simulink model "No_Kalman_FullSystem"  (R2024a)
settings: Solver=FixedStepAuto  StartTime=0.0  StopTime=0.05  FixedStep=0.05  RelTol=1e-3
model workspace (MAT data in the model file):
  Delta_t = 0.1
  J1 = 0.833333333333
  J2 = 1.08333333333
  J3 = 0.416666666667
  NoiseCov = [0.5  0  0  0  0  0  0; 0  0.5  0  0  0  0  0; 0  0  0.5  0  0  0  0; 0  0  0  0.5  0  0  0; 0  0  0  0  0.5  0  0; 0  0  0  0  0  0.5  0; 0  0  0  0  0  0  0.5]
  Orbit_Incl = 51.6
  Q_identity = [0.05  0  0  0  0  0  0; 0  0.05  0  0  0  0  0; 0  0  0.05  0  0  0  0; 0  0  0  0.05  0  0  0; 0  0  0  0  0.05  0  0; 0  0  0  0  0  0.05  0; 0  0  0  0  0  0  0.05]
  Sig = Simulink.Signal
  Sig.DataType = 'auto'
  Sig.Dimensions = -1
  Sig.DimensionsMode = 'auto'
  Sig.Complexity = 'auto'
  Sig.SampleTime = -1
  Sig.SamplingMode = 'auto'
  controlRun = 1
  jd_input = 2458850.00006
  m = 100
  n = 7
  prev_torque_input = [-0.00050779436613; -0.000537657150204; 0.000673104501962]
  q_ff_in = [0.768162333731 -0.000607721012165 0.00073835510125 -0.64025441392]
  s_input = [0.126195549094  -0.0456814887308  -0.161020672839  -0.0555064713506  -0.000532606081941  0.000213749478451  -0.00066383496662; -0.0456814887308  0.0300852731757  0.0643242310821  0.0221411903621  0.000189759589489  -0.00017191746789  0.000231570257692; -0.161020672839  0.0643242310821  0.23849220968  0.0781228177648  0.000857803282785  -0.000316346290687  0.000810872548691; -0.0555064713506  0.0221411903621  0.0781228177648  0.0387660028181  0.000267247923751  -0.000128314700029  0.000266373914183; -0.000532606081941  0.000189759589489  0.000857803282785  0.000267247923751  0.0414168924362  -1.57036491515e-05  2.42567511858e-05; 0.000213749478451  -0.00017191746789  -0.000316346290687  -0.000128314700029  -1.57036491515e-05  0.0414098493382  -0.000222921548759; -0.00066383496662  0.000231570257692  0.000810872548691  0.000266373914183  2.42567511858e-05  -0.000222921548759  0.0414237557466]
  s_input_cons = [1.94870414  1.25588909  1.4416761  1.0780205  1.49168854  1.53894753  1.37981514; 1.25588909  2.30599344  1.57766712  1.62980068  1.46050557  1.31460547  1.13813509; 1.4416761  1.57766712  1.70958392  1.12140846  1.38322267  1.58836736  1.34392315; 1.0780205  1.62980068  1.12140846  1.77837393  1.21690337  0.94427956  1.46043147; 1.49168854  1.46050557  1.38322267  1.21690337  2.06327445  1.39185931  1.33424815; 1.53894753  1.31460547  1.58836736  0.94427956  1.39185931  2.02772691  1.7277207; 1.37981514  1.13813509  1.34392315  1.46043147  1.33424815  1.7277207  2.16380015]
  savedTorque = [-0.000405741986708; 0.000253632743324; 0.00087809103841]
  t_step = 0.05
  v_icrf_input = [-2750.79951667 6666.40019935 2573.40073342]
  x_icrf_input = [3649696.21765 3308209.1663 -4676596.46157]
  x_icrf_input_cons = [3649700 3308200 -4676600]
  x_input = [-0.400194557056; -0.190242708716; -0.896104173464; -0.0254821228337; 0.443902714712; -0.277487336755; -0.960677002834]
  x_input_cons = [0.2; 0.6; 0.5; 0.59160797831; 0.1; 0.4; 0.9]
libraries: aerolibsatdyn x1, aerolibtransform2 x1, aerolibutil x1
settings Model: Creator=alenachan  LastModifiedBy=ruimi

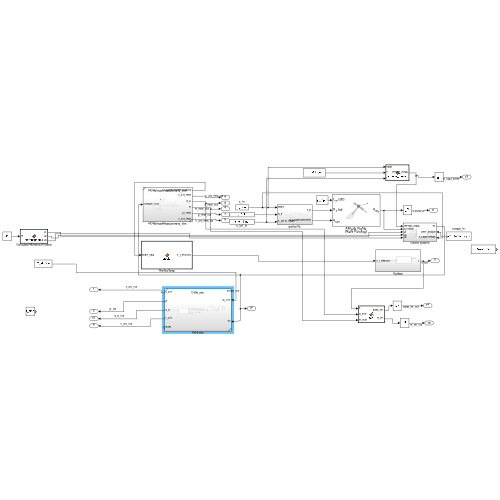
[thumbnail: Simulink's stored preview of the top-level diagram]
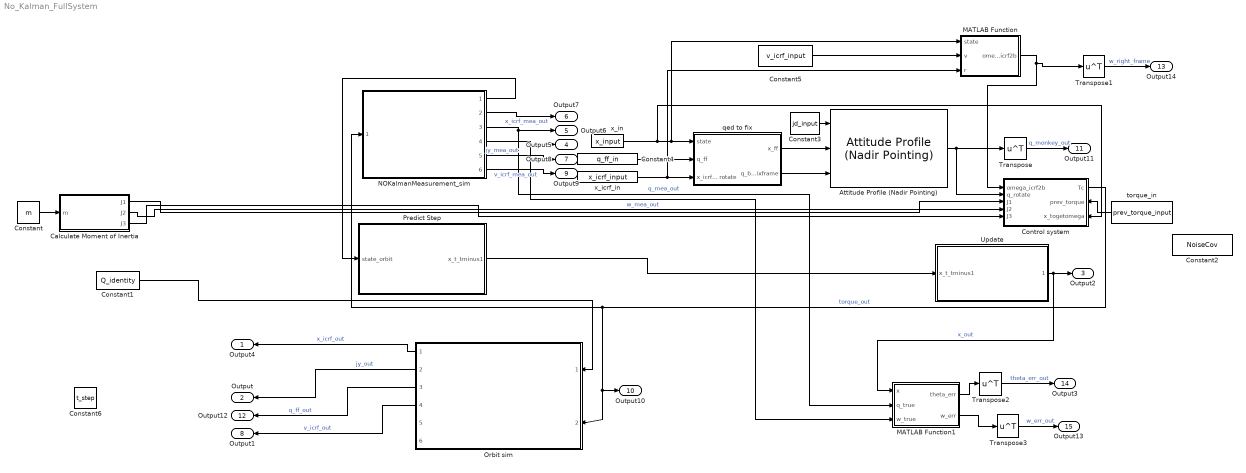
== system No_Kalman_FullSystem ==
  " Calculate Moment of Inertia" : MATLAB Function  Priority=10  TreatAsAtomicUnit=on
  Attitude Profile (Nadir Pointing) : aerolibsatdyn/Attitude Profile (Nadir Pointing)  Priority=3  outputError=on  outputFinalAttitude=off  portFrame=Fixed-frame  pointingMode=Point at nadir  celestialTarget=Sun  tunablePointing=off  primaryAlignmentSrc=Dialog  primaryAlignment=[0 0 1]  secondaryAlignmentSrc=Dialog  secondaryAlignment=[1 0 0]  constraintFrame=ICRF  primaryConstraintSrc=Dialog  primaryConstraint=[1 0 0]  secondaryConstraintSrc=Dialog  secondaryConstraint=[0 1 0]
  Constant : Constant  Value=m
  Constant1 : Constant  Value=Q_identity
  Constant2 : Constant  Value=NoiseCov
  Constant3 : Constant  Value=jd_input
  Constant4 : Constant  Value=q_ff_in
  Constant5 : Constant  Value=v_icrf_input
  Constant6 : Constant  Value=t_step
  Control system : Subsystem  Priority=4
      settings: PortSchema="{\"entries\":[{\"content\":{\"sides\":[{\"content\":{\"connectorIds\":[\"In1\",\"In2\",\"In3\",\"In4\",\"In5\"]},\"type\":\"ConnectorPlacement.EquallySpacedRectSide\",\"uuid\":\"8eb5f269-cc65-4267-936a-9f0f4ccd4d18\"},{\"content\":{\"connectorIds\":[\"Out1\",\"In6\",\"In7\"],\"side\":\"RIGHT\"},\"type\":\"ConnectorPlacement.EquallySpacedRectSide\",\"uuid\":\"3df96c14-e4ae-45ba-8fc0-de3a9fdcf55a\"},{\"content\":{\"side\":\"TOP\"},\"type\":\"ConnectorPlacement.EquallySpacedRectSide\",\"uuid\":\"e3effbcc-2fcc-4dea-811c-5aa639521533\"}]},\"type\":\"ConnectorPlacement.EquallySpacedConnector\",\"uuid\":\"93bbc224-b85a-4291-8bf8-2645c40efc9b\"}],\"packageUris\":[\"http://schema.mathworks.com/mf0/Connector/R2020b\"],\"version\":\"1.0\"}"
  MATLAB Function : MATLAB Function  TreatAsAtomicUnit=on
  MATLAB Function1 : MATLAB Function  TreatAsAtomicUnit=on
  NOKalmanMeasurement_sim : Subsystem  ReferencedSubsystem=NOKalmanMeasurement_sim
  Orbit sim : Subsystem  Priority=7  ReferencedSubsystem=Orbit_sim
  Predict Step : MATLAB Function  Priority=11  TreatAsAtomicUnit=on
  Transpose{,1..3} (4 alike) : Math  Operator=transpose
  Update : Subsystem  Priority=12
  qed to fix : Subsystem  Priority=2
  torque_in : Constant  Value=prev_torque_input
  x_icrf_in : Constant  Value=x_icrf_input
  x_in : Constant  Value=x_input
  Output4 : Outport
  Output : Outport  Port=2
  Output2 : Outport  Port=3
  Output5 : Outport  Port=4
  Output6 : Outport  Port=5
  Output7 : Outport  Port=6
  Output8 : Outport  Port=7
  Output1 : Outport  Port=8
  Output9 : Outport  Port=9
  Output10 : Outport  Port=10
  Output11 : Outport  Port=11
  Output12 : Outport  Port=12
  Output14 : Outport  Port=13
  Output3 : Outport  Port=14
  Output13 : Outport  Port=15
  wires:
  Control system/1(Tc) -> NOKalmanMeasurement_sim/1, Output10/1, Orbit sim/2  "torque_out"
  Orbit sim/2 -> Output/1  "jy_out"
  Orbit sim/1 -> Output4/1  "x_icrf_out"
  Constant/1 -> " Calculate Moment of Inertia"/1(m)
  " Calculate Moment of Inertia"/1(J1) -> Control system/3(J1)
  " Calculate Moment of Inertia"/2(J2) -> Control system/4(J2)
  " Calculate Moment of Inertia"/3(J3) -> Control system/5(J3)
  Constant1/1 -> Orbit sim/1
  x_in/1 -> Control system/7(x_togetomega), MATLAB Function/1(state), qed to fix/1(state)
  x_icrf_in/1 -> MATLAB Function/3(r), qed to fix/3(x_icrf to rotate)
  Predict Step/1(x_t_tminus1) -> Update/1(x_t_tminus1)
  Update/1(1) -> MATLAB Function1/1(x), Output2/1  "x_out"
  Orbit sim/3 -> Output12/1  "q_ff_out"
  NOKalmanMeasurement_sim/4 -> MATLAB Function1/3(w_true), Output5/1  "w_mea_out"
  NOKalmanMeasurement_sim/3 -> MATLAB Function1/2(q_true), Output6/1  "q_mea_out"
  NOKalmanMeasurement_sim/2 -> Output7/1  "x_icrf_mea_out"
  NOKalmanMeasurement_sim/5 -> Output8/1  "jy_mea_out"
  Orbit sim/4 -> Output1/1  "v_icrf_out"
  NOKalmanMeasurement_sim/6 -> Output9/1  "v_icrf_mea_out"
  torque_in/1 -> Control system/6(prev_torque)
  Transpose/1 -> Output11/1  "q_monkey_out"
  Constant3/1 -> Attitude Profile (Nadir Pointing)/1
  qed to fix/2(q_bodyToFixframe) -> Attitude Profile (Nadir Pointing)/3
  Constant4/1 -> qed to fix/2(q_ff)
  qed to fix/1(x_ff) -> Attitude Profile (Nadir Pointing)/2
  Attitude Profile (Nadir Pointing)/1 -> Transpose/1, Control system/2(q_rotate)
  Constant5/1 -> MATLAB Function/2(v)
  MATLAB Function/1(omega_icrf2b) -> Transpose1/1, Control system/1(omega_icrf2b)
  Transpose1/1 -> Output14/1  "w_right_frame"
  NOKalmanMeasurement_sim/1 -> Predict Step/1(state_orbit)
  MATLAB Function1/1(theta_err) -> Transpose2/1
  Transpose2/1 -> Output3/1  "theta_err_out"
  MATLAB Function1/2(w_err) -> Transpose3/1
  Transpose3/1 -> Output13/1  "w_err_out"

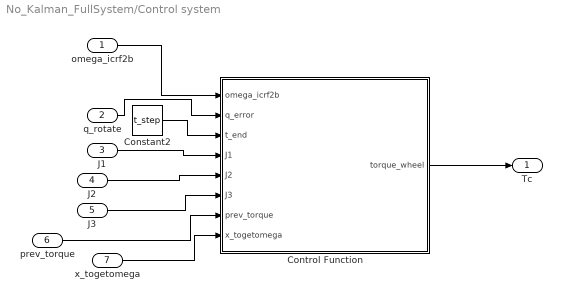
== system No_Kalman_FullSystem/Control system ==
  omega_icrf2b : Inport
  q_rotate : Inport  Port=2
  J1 : Inport  Port=3
  J2 : Inport  Port=4
  J3 : Inport  Port=5
  prev_torque : Inport  Port=6
  x_togetomega : Inport  Port=7
  Constant2 : Constant  Value=t_step
  Control Function : MATLAB Function  TreatAsAtomicUnit=on
  Tc : Outport
  wires:
  Constant2/1 -> Control Function/3(t_end)
  Control Function/1(torque_wheel) -> Tc/1
  q_rotate/1 -> Control Function/2(q_error)
  J1/1 -> Control Function/4(J1)
  J2/1 -> Control Function/5(J2)
  J3/1 -> Control Function/6(J3)
  prev_torque/1 -> Control Function/7(prev_torque)
  x_togetomega/1 -> Control Function/8(x_togetomega)
  omega_icrf2b/1 -> Control Function/1(omega_icrf2b)

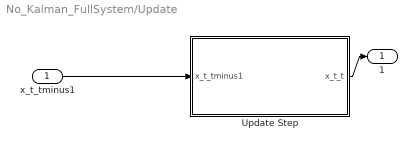
== system No_Kalman_FullSystem/Update ==
  x_t_tminus1 : Inport
  Update Step : MATLAB Function  TreatAsAtomicUnit=on
  1 : Outport
  wires:
  x_t_tminus1/1 -> Update Step/1(x_t_tminus1)
  Update Step/1(x_t_t) -> 1/1

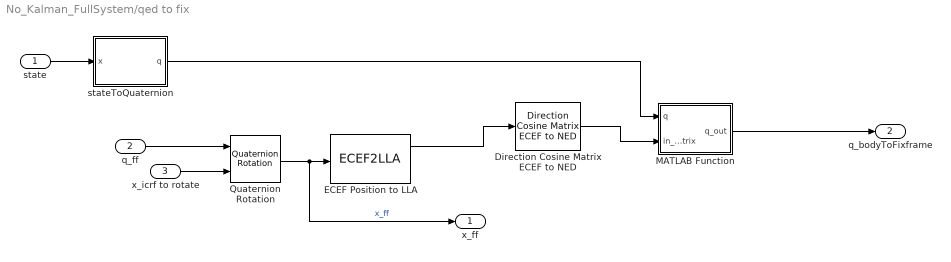
== system No_Kalman_FullSystem/qed to fix ==
  state : Inport
  q_ff : Inport  Port=2
  x_icrf to rotate : Inport  Port=3
  Direction Cosine Matrix ECEF to NED : aerolibtransform2/Direction Cosine Matrix ECEF to NED
  ECEF Position to LLA : ECEF2LLA
  MATLAB Function : MATLAB Function  TreatAsAtomicUnit=on
  Quaternion Rotation : aerolibutil/Quaternion Rotation
  stateToQuaternion : MATLAB Function  TreatAsAtomicUnit=on
  x_ff : Outport
  q_bodyToFixframe : Outport  Port=2
  wires:
  state/1 -> stateToQuaternion/1(x)
  Quaternion Rotation/1 -> x_ff/1, ECEF Position to LLA/1  "x_ff"
  x_icrf to rotate/1 -> Quaternion Rotation/2
  ECEF Position to LLA/1 -> Direction Cosine Matrix ECEF to NED/1
  Direction Cosine Matrix ECEF to NED/1 -> MATLAB Function/2(in_matrix)
  stateToQuaternion/1(q) -> MATLAB Function/1(q)
  MATLAB Function/1(q_out) -> q_bodyToFixframe/1
  q_ff/1 -> Quaternion Rotation/1

== matlab function No_Kalman_FullSystem/Update/Update Step ==
  data: x_t_tminus1 input; x_t_t output
function x_t_t  = update(x_t_tminus1)

%Update
x_t_t = x_t_tminus1;
x_t_t(1:4)=x_t_t(1:4)/norm(x_t_t(1:4));

end

== matlab function No_Kalman_FullSystem/Predict Step ==
  data: state_orbit input; x_t_tminus1 output
function x_t_tminus1 = predict(state_orbit)


x_t_tminus1 = state_orbit; %use state from orbit with noise
% x_t_tminus1 = feval(f_t,x_tminus1_tminus1);

== matlab function No_Kalman_FullSystem/qed to fix/MATLAB Function ==
  data: q input; in_matrix input; q_out output
function q_out= fcn(q, in_matrix)
inv_m = inv(in_matrix);
q_second = rotm2quat(inv_m);
q_first = quatconj(q);
q_out = transpose(quatmultiply(q_second,q_first));

== matlab function No_Kalman_FullSystem/qed to fix/stateToQuaternion ==
  data: x input; q output
function q = getq(x)
q_temp = x(1:4);
q = transpose(q_temp);
end

== matlab function No_Kalman_FullSystem/MATLAB Function1 ==
  data: x input; theta_err output; q_true input; w_true input; w_err output
function [theta_err, w_err]= fcn(x, q_true, w_true)
theta_est = 2*acos(x(1));
theta_true = 2*acos(q_true(1));
theta_err = theta_est - theta_true;

w_err = transpose(x(5:7))-w_true;

== matlab function No_Kalman_FullSystem/MATLAB Function ==
  data: state input; v input; omega_icrf2b output; r input
function omega_icrf2b = omega_frame(state,v,r)
omega_ned2b = state(5:7);
omega_icrf2ned = -cross(r,v)/norm(r)^2;
omega_icrf2b = omega_ned2b + omega_icrf2ned;

== matlab function No_Kalman_FullSystem/ Calculate Moment of Inertia ==
  data: m input; J1 output; J2 output; J3 output
function [J1,J2,J3]=momentInertia(m)
J1 = m/120;
J2 = 13*m/1200;
J3 = 5*m/1200;
coder.extrinsic("get_param");
mdlWks = get_param('No_Kalman_FullSystem','ModelWorkspace');
assignin(mdlWks,"J1",J1)
assignin(mdlWks,"J2",J2)
assignin(mdlWks,"J3",J3)
end

== matlab function No_Kalman_FullSystem/Control system/Control Function ==
  data: omega_icrf2b input; q_error input; t_end input; torque_wheel output size=[3 1]; J1 input; J2 input; J3 input; prev_torque input; x_togetomega input
function torque_wheel = fcn(omega_icrf2b, q_error, t_end, J1, J2, J3, prev_torque, x_togetomega)
coder.extrinsic("get_param");
coder.extrinsic("getVariable");
coder.extrinsic("quat2angle");

mdlWks = get_param('No_Kalman_FullSystem','ModelWorkspace');
ctrlRn = getVariable(mdlWks,'controlRun');
if ~ctrlRn
    %disp('enter Control');

    if(norm(x_togetomega(5:7)) > 0.15)
        torque_wheel_calc = -0.8*x_togetomega(5:7);
    else
        theta = abs(2*acos(q_error(1))); % magnitude
        direction = [q_error(2);q_error(3); q_error(4)]/abs(sin(theta/2)); %3d-vector
        omega_cur_indir=dot(omega_icrf2b*t_end,direction);
        acc = ((theta - omega_cur_indir*t_end)* 2)/(t_end^2); % magnitude
        acc_directed = acc*direction; %3d-vector
        
        I_sate = [J1,0,0; 0,J2,0; 0,0,J3]; % define moment of inertia (same for every wheel)
        torque_wheel_calc = 0.9*I_sate * acc_directed + 0.1*prev_torque; % 3-d vector; 0.1 is momentum coefficient
    end

    max_torque = .001; % 0.824 * 10^(-2); %reasonable estimate from CSI document
    if norm(torque_wheel_calc) > max_torque % scale to maximum allowed magnitude
        % disp("Torque is beyond physical limit.");
        torque_wheel = (max_torque/norm(torque_wheel_calc))* torque_wheel_calc;
    else
        torque_wheel = torque_wheel_calc;
    end

    assignin(mdlWks,'savedTorque', torque_wheel);
    assignin(mdlWks,'controlRun', true);    
else
    %disp('skipped control');
    torque_wheel = getVariable(mdlWks,'savedTorque'); % this ensures that value doesn't zero out after multiple runs
end
